simulink model "pidbonuocroirac"  (Simulink 9.3)
settings: Solver=FixedStepAuto  StartTime=0.0  StopTime=200  FixedStep=0.1  RelTol=1e-3
values from neighbouring files (symbols this model uses):
  a = 1    [thongsohethong.m]
  Amax = 200    [thongsohethong.m]
  Amin = 100    [thongsohethong.m]
  CD = 0.6    [thongsohethong.m]
  h_init = 0    [thongsohethong.m]
  hmax = 50    [thongsohethong.m]
  k = 300    [thongsohethong.m]
  Kd = 0.1    [thongsohethong.m]
  Ki = 0.01    [thongsohethong.m]
  Kp = 5    [thongsohethong.m]
undefined symbols (not defined in the file or in its folder): DiscIntNeverNeededParam
libraries: simulink x1
settings Model: Creator=TDNhon  LastModifiedBy=TDNhon
settings DataIOCC: SaveFormat=Dataset  SignalLoggingSaveFormat=Dataset  ReturnWorkspaceOutputs=on
settings OptimizationCC: LifeSpan=auto
settings DebuggingCC: UnderspecifiedInitializationDetection=Simplified  MergeDetectMultiDrivingBlocksExec=error  FcnCallInpInsideContextMsg=error  SFUnexpectedBacktrackingDiag=error  SFNoUnconditionalDefaultTransitionDiag=error  SFExecutionAtInitializationDiag=warning  ArithmeticOperatorsInVariantConditions=error
settings HardwareCC: ProdBitPerPointer=64  ProdBitPerSizeT=64  ProdBitPerPtrDiffT=64  ProdLargestAtomicFloat=Float  ProdIntDivRoundTo=Zero  ProdEndianess=LittleEndian  ProdWordSize=64  ProdHWDeviceType=Intel->x86-64 (Windows64)
settings ModelReferenceCC: PropagateSignalLabelsOutOfModel=on
settings SFSimCC: SimUseLocalCustomCode=on
settings RTWCC: RTWUseLocalCustomCode=on
settings CodeAppCC: StateflowObjectComments=off
settings GRTTargetCC: TargetLangStandard=C99 (ISO)  CombineOutputUpdateFcns=on  GRTInterface=off
settings ConfigComp: CovMetricSettings=dwe  CovHtmlReporting=off  CovSaveCumulativeToWorkspaceVar=off  CovSaveSingleToWorkspaceVar=off  CovExternalEMLEnable=on

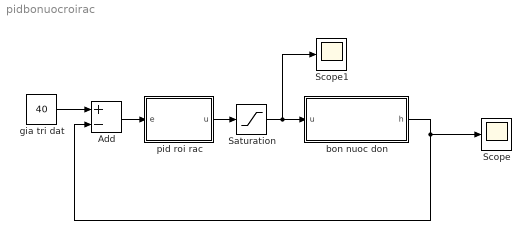
== system pidbonuocroirac ==
  Add : Sum  Inputs=+-
  Saturation : Saturate  UpperLimit=12  LowerLimit=0
  Scope : Scope
  Scope1 : Scope
  bon nuoc don : Subsystem
  gia tri dat : Constant  Value=40
  pid roi rac : Subsystem
  wires:
  gia tri dat/1 -> Add/1
  bon nuoc don/1(h) -> Scope/1, Add/2
  Add/1 -> pid roi rac/1(e)
  pid roi rac/1("u ") -> Saturation/1
  Saturation/1 -> Scope1/1, bon nuoc don/1(u)

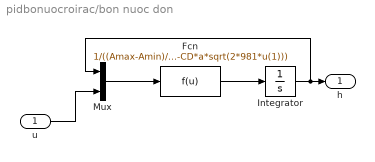
== system pidbonuocroirac/bon nuoc don ==
  u : Inport
  Fcn : Fcn  Expr=1/((Amax-Amin)/hmax*u(1)+Amin)*(k*u(2)-CD*a*sqrt(2*981*u(1)))
  Integrator : Integrator  InitialCondition=h_init
  Mux : Mux  Inputs=2
  h : Outport
  wires:
  Integrator/1 -> Mux/1, h/1
  Fcn/1 -> Integrator/1
  u/1 -> Mux/2
  Mux/1 -> Fcn/1

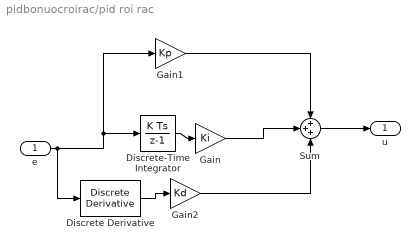
== system pidbonuocroirac/pid roi rac ==
  e : Inport
  Discrete Derivative : simulink/Discrete/Discrete Derivative  gainval=1.0  ICPrevScaledInput=0.0  OutMin=[]  OutMax=[]  OutDataType=fixdt(1, 16)  OutScaling=2^-10  DoSatur=off
  Discrete-Time Integrator : DiscreteIntegrator  SampleTime=-1  ICPrevOutput=DiscIntNeverNeededParam  ICPrevScaledInput=DiscIntNeverNeededParam
  Gain : Gain  Gain=Ki
  Gain1 : Gain  Gain=Kp
  Gain2 : Gain  Gain=Kd
  Sum : Sum  Inputs=+++
  "u " : Outport
  wires:
  e/1 -> Discrete Derivative/1, Discrete-Time Integrator/1, Gain1/1
  Discrete-Time Integrator/1 -> Gain/1
  Discrete Derivative/1 -> Gain2/1
  Gain1/1 -> Sum/1
  Gain/1 -> Sum/2
  Gain2/1 -> Sum/3
  Sum/1 -> "u "/1
